simulink model "lavadora_industrial_2niveles"  (R2015b)
settings: Solver=VariableStepAuto  StartTime=0.0  StopTime=10.0  RelTol=1e-3
undefined symbols (not defined in the file): p5_nivel1, p5_nivel2
libraries: fuzblock x2
settings Model: Creator=Fabian  LastModifiedBy=Fabian

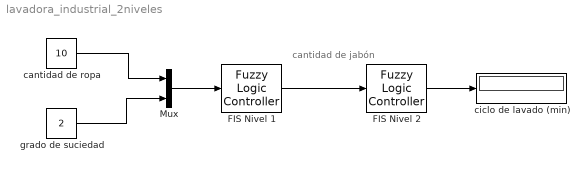
== system lavadora_industrial_2niveles ==
  note: cantidad de
      | jabón
  FIS Nivel 1 : fuzblock/Fuzzy Logic  Controller  fis=[p5_nivel1]
  FIS Nivel 2 : fuzblock/Fuzzy Logic  Controller  fis=[p5_nivel2]
  Mux : Mux  Inputs=2
  cantidad de ropa : Constant  Value=10
  ciclo de lavado (min) : Display
  grado de suciedad : Constant  Value=2
  wires:
  cantidad de ropa/1 -> Mux/1
  grado de suciedad/1 -> Mux/2
  Mux/1 -> FIS Nivel 1/1
  FIS Nivel 1/1 -> FIS Nivel 2/1
  FIS Nivel 2/1 -> ciclo de lavado (min)/1
